simulink model "PMSM_FOC_Tractio"  (R2019b)
settings: Solver=FixedStepAuto  StartTime=0.0  StopTime=10  RelTol=1e-3
model workspace (MAT data in the model file):
  wc = Simulink.Parameter
  wc.DataType = 'auto'
  wc.Dimensions = [0 0]
values from neighbouring files (symbols this model uses):
  Cosine_table = 1.0 0.99999529 0.99999058 0.99998587 0.99998116 0.99996704 0.99995291 0.99993885 0.99992472 0.99990118 0.99987763 0.99985409 0.9998306 0.99979764 0.99976468 0.99973178 0.99969882 0.99965644 0.99961412 0.99957174 0.99952942 0.99947762 0.99942589 0.99937415 0.99932235 0.9992612 0.99920005 0.99913889 0.99907768 0.99900717 0.99893659 0.99886602 0.99879545 0.99871546 0.99863547 0.99855554 0.99847555 0.    [Hall_HFI_FOC_Data.sldd]
  Flux = 0.00529276    [Hall_HFI_FOC_Data.sldd]
  MTPA_id_table = 0.22889 0.23462678 0.23770036 0.2381243 0.23591207 0.23107713 0.2236329 0.21359272 0.20096992 0.18577772 0.16802935 0.14773798 0.12491672 0.099578641 0.071736768 0.041404068 0.0085934745 -0.026682133 -0.064409919 -0.10457709 -0.14717092 -0.1921787 -0.2395878 -0.28938559 -0.34155953 -0.39609709 -0.45298585 -0.51221335 -0.57376724 -0.63763517 -0.70380485 -0.77226412 -0.84300071 -0.91600245 -0.991257    [Hall_HFI_FOC_Data.sldd]
  MTPA_iq_table = -1.0417 -0.16083497 0.71926296 1.5985928 2.4771533 3.3549435 4.2319627 5.1082091 5.9836826 6.8583813 7.732305 8.6054525 9.4778223 10.349415 11.220228 12.090261 12.959513 13.827983 14.69567 15.562573 16.428694 17.294027 18.158575 19.022335 19.885307 20.747492 21.608887 22.469492 23.329306 24.188328 25.046556 25.903992 26.760633 27.616482 28.471533 29.325788 30.179247 31.031908 31.883772 32.734837 3    [Hall_HFI_FOC_Data.sldd]
  MTPA_Te_Max = 800.0    [Hall_HFI_FOC_Data.sldd]
  MTPA_Te_Min = 0.0    [Hall_HFI_FOC_Data.sldd]
  Sine_table = 0.0 0.0015339879 0.0030679768 0.0046019657 0.0061359555 0.0076698866 0.0092038177 0.010737749 0.012271681 0.013805497 0.015339312 0.016873131 0.018406944 0.019940587 0.021474229 0.023007872 0.024541514 0.026074925 0.027608337 0.029141748 0.03067516 0.032208283 0.033741407 0.035274528 0.036807653 0.038340431 0.039873205 0.04140598 0.042938754 0.04447113 0.046003502 0.047535874 0.049068246 0.0506001    [Hall_HFI_FOC_Data.sldd]
undefined symbols (not defined in the file or in its folder): CL_Param, ctrlParamsPI, DiscIntNeverNeededParam, Flux_weak, HFI, inverter, magnitude, OPL_Param, pmsm, sigbuilder_block, SMO, SVPWM
libraries: powerlib x22, fl_lib x18, simulink x7, nesl_utility x7, powerlib_meascontrol x3, dspstat3 x3, powerlib_extras x1, ee_lib x1
(part 1 of 4)
settings Model: Creator=jt  LastModifiedBy=Administrator
settings DataIOCC: LimitDataPoints=on  SaveFormat=Array  ReturnWorkspaceOutputs=off
settings OptimizationCC: DefaultParameterBehavior=Inlined  UseDivisionForNetSlopeComputation=on  GainParamInheritBuiltInType=on  UseFloatMulNetSlope=on  InlineInvariantSignals=on  PassReuseOutputArgsAs=Individual arguments  ZeroExternalMemoryAtStartup=off  ZeroInternalMemoryAtStartup=off  NoFixptDivByZeroProtection=on  EfficientFloat2IntCast=on  LifeSpan=1  OptimizeBlockOrder=speed  DifferentSizesBufferReuse=on  EfficientTunableParamExpr=on
settings DebuggingCC: AlgebraicLoopMsg=none  MaxConsecutiveZCsMsg=none  SolverPrmCheckMsg=warning  ParameterTunabilityLossMsg=error  AllowSymbolicDim=off  SFUnexpectedBacktrackingDiag=warning  SFNoUnconditionalDefaultTransitionDiag=warning  SFExecutionAtInitializationDiag=none  ArithmeticOperatorsInVariantConditions=warning
settings HardwareCC: ProdBitPerPointer=32  ProdBitPerSizeT=32  ProdBitPerPtrDiffT=32  ProdLargestAtomicInteger=Long  ProdLargestAtomicFloat=Double  ProdEndianess=BigEndian  ProdWordSize=32  ProdLongLongMode=on  ProdHWDeviceType=Freescale->32-bit PowerPC
settings ModelReferenceCC: PropagateSignalLabelsOutOfModel=off
settings SFSimCC: SimUseLocalCustomCode=off  SimParseCustomCode=off  MATLABDynamicMemAlloc=off  CustomCodeUndefinedFunction=UseInterfaceOnly
settings RTWCC: SystemTargetFile=ert.tlc  GenCodeOnly=on  TemplateMakefile=ert_default_tmf  GenerateReport=on  RTWUseLocalCustomCode=off  IncludeHyperlinkInReport=on  LaunchReport=on  GenerateTraceInfo=on  GenerateTraceReport=on  GenerateTraceReportSl=on  GenerateTraceReportSf=on  GenerateTraceReportEml=on  GenerateCodeMetricsReport=on
settings CodeAppCC: ForceParamTrailComments=on  IgnoreCustomStorageClasses=off  OperatorAnnotations=on  SimulinkDataObjDesc=on  SFDataObjDesc=on  CustomSymbolStrGlobalVar=rt$N$M  CustomSymbolStrType=$N$M  CustomSymbolStrFcn=$N$M$F  CustomSymbolStrMacro=$N$M  InsertBlockDesc=on
settings ERTTargetCC: GenerateSampleERTMain=on  IncludeMdlTerminateFcn=off  CombineSignalStateStructs=on  SupportNonInlinedSFcns=on  InlinedParameterPlacement=NonHierarchical  ERTCustomFileTemplate=example_file_process.tlc
settings ConfigComp: CovMetricSettings=dw  CovHtmlReporting=on  CovSaveCumulativeToWorkspaceVar=on  CovSaveSingleToWorkspaceVar=on  CovExternalEMLEnable=off  CovSFcnEnable=off
settings SimscapeCC: SimscapeNormalizeSystem=off

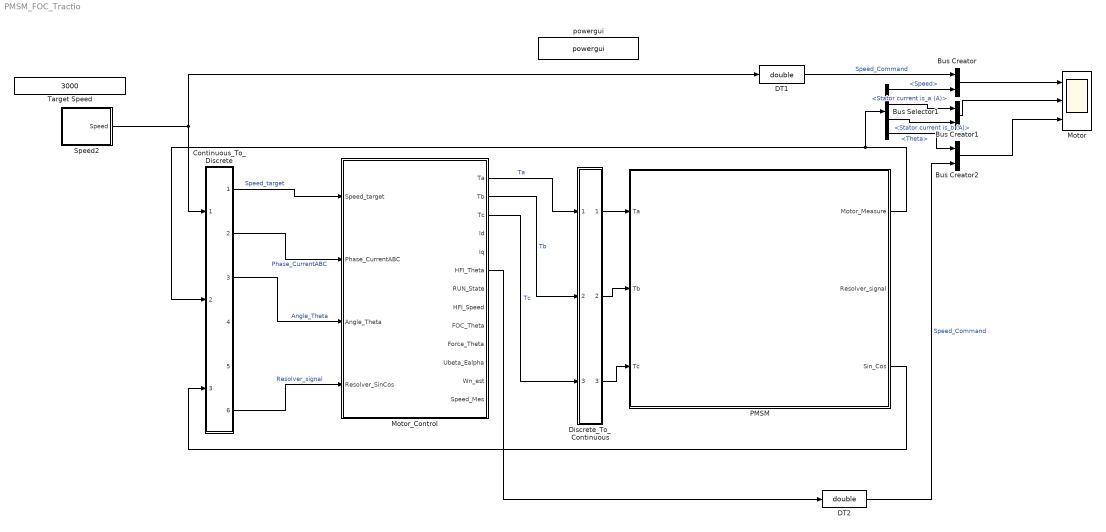
== system PMSM_FOC_Tractio ==
  Bus Creator : BusCreator  Inputs=2
  Bus Creator1 : BusCreator  Inputs=2
  Bus Creator2 : BusCreator  Inputs=2
  Bus Selector1 : BusSelector  OutputSignals=Speed,Stator current is_a (A),Stator current is_b (A),Theta
  Continuous_To_Discrete : Subsystem
      mask Display: fprintf('C/D')
  DT1 : DataTypeConversion  OutDataTypeStr=double
  DT2 : DataTypeConversion  OutDataTypeStr=double
  Discrete_To_Continuous : Subsystem  Description=""
      mask Display: fprintf('D/C')
  Motor : Scope  NumInputPorts=3
  Motor_Control : Subsystem  TreatAsAtomicUnit=on
  PMSM : Subsystem
      mask Display: image('$imagefile'); % Use "Edit Image" on toolstrip to change.
  Speed2 : Subsystem  Tag=STV Subsys  LoadFcn=sigbuilder_block('load');  StartFcn=sigbuilder_block('start');  StopFcn=sigbuilder_block('stop');  ClipboardFcn=sigbuilder_block('clipboard');  mask(Sigbuilder block){tuvar=[0:10]}
      mask help: Simulink:masks:SigbuilderBlock_MD
      mask init:
      | if ~strcmp(get_param(bdroot(gcbh),'SimulationStatus'),'stopped') tuvar = sigbuilder_block('maskInit'); end
      settings: CopyFcn=sigbuilder_block('copy');  DeleteFcn=sigbuilder_block('delete');  ModelCloseFcn=sigbuilder_block('modelClose');  PreSaveFcn=sigbuilder_block('preSave');  PauseFcn=sigbuilder_block('pause');  ContinueFcn=sigbuilder_block('continue');  NameChangeFcn=sigbuilder_block('namechange');  OpenFcn=sigbuilder_block('open',[48.5 0 906 449 ]);  CloseFcn=sigbuilder_block('close');
      mask Display: plot(0, 0, 100, 100,[2, 2, 32, 32, 2], [68, 8, 8, 68, 68],[32, 2], [38, 38], [32, 19, 2],[53, 60, 44], [32, 17, 17, 2],[16, 16, 31, 31]);txt = getActiveGroup(gcbh);text(2, 100, txt,'verticalAlignment', 'top');
  Target Speed : Constant  Value=3000
  powergui : powerlib/powergui  Priority=1  SimulationMode=Discrete  SampleTime=1e-5  frequency=60  Iterations=50  frequencyindice=0  Pbase=100e6  ErrMax=1e-4  UnitsV=kV  UnitsW=MW  buscounter=0  FunctionMessages=off  echomessages=off  EnableUseOfTLC=off  CurrentSourceSwitches=off  DisableSnubberDevices=off  DisableRonSwitches=off  DisableVfSwitches=off  DisplayEquations=off  AutomaticDiscreteSolvers=off  SolverType=Tustin  Interpol=off  ExternalGateDelay=off  methode=off  Ts=0  x0status=blocks  SPID=off  SwTol=0  HookPort=off  NonlinearTolerance=1e-4  nMaxIteration=100  ContinueOnMaxIteration=off  RestoreLinks=warning  ResistiveCurrentMeasurement=off  Frange=[0:2:500]  Ylog=off  Xlog=on  ShowGrid=off  save=off  variable=ZData  structure=0  ZoomFFT=on  StartTime=0.0  cycles=1  DisplayStyle=1  fundamental=60  FreqAxis=off  MaxFrequency=1000  frequencyindicesteady=1  RmsSteady=1  display=off
      settings: SourceProductName=Simscape Electrical
  wires:
  Discrete_To_Continuous/1(T1) -> PMSM/1(Ta)
  Discrete_To_Continuous/2(T2) -> PMSM/2(Tb)
  Discrete_To_Continuous/3(T3) -> PMSM/3(Tc)
  PMSM/1(Motor_Measure) -> Continuous_To_Discrete/2(Motor_Measurements), Bus Selector1/1
  Continuous_To_Discrete/1(Speed_target) -> Motor_Control/1(Speed_target)  "Speed_target"
  Continuous_To_Discrete/3(Theta) -> Motor_Control/3(Angle_Theta)  "Angle_Theta"
  Motor_Control/1(Ta) -> Discrete_To_Continuous/1(Ta)  "Ta"
  Motor_Control/2(Tb) -> Discrete_To_Continuous/2(Tb)  "Tb"
  Motor_Control/3(Tc) -> Discrete_To_Continuous/3(Tc)  "Tc"
  Bus Selector1/1 -> Bus Creator/2  "<Speed>"
  Bus Creator/1 -> Motor/1
  Bus Selector1/2 -> Bus Creator1/1  "<Stator current is_a (A)>"
  Bus Selector1/3 -> Bus Creator1/2  "<Stator current is_b (A)>"
  Bus Creator1/1 -> Motor/2
  Speed2/1(Speed) -> DT1/1, Continuous_To_Discrete/1(Speed_Command)
  DT1/1 -> Bus Creator/1  "Speed_Command"
  Continuous_To_Discrete/6(Resolver_measured) -> Motor_Control/4(Resolver_SinCos)  "Resolver_signal"
  PMSM/3(Sin_Cos) -> Continuous_To_Discrete/3(Sin_Cos)
  Continuous_To_Discrete/2(Phase_CurrentABC) -> Motor_Control/2(Phase_CurrentABC)  "Phase_CurrentABC"
  Bus Selector1/4 -> Bus Creator2/1  "<Theta>"
  Motor_Control/6(HFI_Theta) -> DT2/1
  Bus Creator2/1 -> Motor/3
  DT2/1 -> Bus Creator2/2  "Speed_Command"

== system PMSM_FOC_Tractio/Continuous_To_Discrete ==
  note: Continuous To Discrete
  Speed_Command : Inport
  Motor_Measurements : Inport  Port=2
  Sin_Cos : Inport  Port=3
  Bus Selector1 : BusSelector  OutputSignals=Speed,Stator current is_a (A),Stator current is_b (A),Stator current is_c (A),Theta,Vabc
  Bus Selector2 : BusSelector  OutputSignals=Sin,Cos
  DT{1..6} (6 alike) : DataTypeConversion  OutDataTypeStr=single
  Mux1 : Mux  Inputs=2
  Mux2 : Mux  Inputs=3
  RT{1..5} (5 alike) : RateTransition  Integrity=off
  RT6 : RateTransition  Integrity=off  OutPortSampleTime=inverter.Ts
  Speed_target : Outport
  Phase_CurrentABC : Outport  Port=2  PortDimensions=3
  Theta : Outport  Port=3
  Vabc : Outport  Port=4
  Speed_val : Outport  Port=5
  Resolver_measured : Outport  Port=6
  wires:
  DT2/1 -> Speed_val/1  "Speed_Measure"
  DT1/1 -> Speed_target/1  "Speed_Command"
  RT2/1 -> DT2/1
  RT1/1 -> DT1/1
  RT3/1 -> DT3/1
  Motor_Measurements/1 -> Bus Selector1/1
  Speed_Command/1 -> RT1/1
  RT4/1 -> DT4/1
  DT4/1 -> Theta/1  "Theta_Angle"
  Bus Selector1/1 -> RT2/1  "<Speed>"
  Bus Selector1/5 -> RT4/1  "<Theta>"
  DT5/1 -> Vabc/1  "Vabc"
  RT5/1 -> DT5/1
  Bus Selector1/6 -> RT5/1  "<Vabc>"
  DT6/1 -> Resolver_measured/1  "Resolver"
  Sin_Cos/1 -> Bus Selector2/1
  Bus Selector2/1 -> Mux1/1  "<Sin>"
  Bus Selector2/2 -> Mux1/2  "<Cos>"
  Mux1/1 -> RT6/1
  RT6/1 -> DT6/1
  Bus Selector1/2 -> Mux2/1  "<Stator current is_a (A)>"
  Bus Selector1/4 -> Mux2/3  "<Stator current is_c (A)>"
  Bus Selector1/3 -> Mux2/2  "<Stator current is_b (A)>"
  Mux2/1 -> RT3/1
  DT3/1 -> Phase_CurrentABC/1  "Phase_CurrentABC"

== system PMSM_FOC_Tractio/Discrete_To_Continuous ==
  note: Discrete To Continuous
  Ta : Inport
  Tb : Inport  Port=2
  Tc : Inport  Port=3
  DT : DataTypeConversion
  DT1 : DataTypeConversion
  DT2 : DataTypeConversion
  RT : RateTransition  Integrity=off
  RT1 : RateTransition  Integrity=off
  RT2 : RateTransition  Integrity=off
  T1 : Outport
  T2 : Outport  Port=2
  T3 : Outport  Port=3
  wires:
  DT/1 -> RT/1
  Ta/1 -> DT/1  "Tabc"
  DT1/1 -> RT1/1
  Tb/1 -> DT1/1  "Tabc"
  DT2/1 -> RT2/1
  Tc/1 -> DT2/1  "Tabc"
  RT/1 -> T1/1  "Tabc"
  RT1/1 -> T2/1  "Tabc"
  RT2/1 -> T3/1  "Tabc"

== system PMSM_FOC_Tractio/Motor_Control ==
  Speed_target : Inport
  Phase_CurrentABC : Inport  Port=2  PortDimensions=3
  Angle_Theta : Inport  Port=3  OutMin=0  OutMax=2*pi
  Resolver_SinCos : Inport  Port=4  OutMin=0  OutMax=2*pi
  Motor_Control_Funtion : Subsystem
  Ta : Outport
  Tb : Outport  Port=2
  Tc : Outport  Port=3
  Id : Outport  Port=4
  Iq : Outport  Port=5
  HFI_Theta : Outport  Port=6
  RUN_State : Outport  Port=7
  HFI_Speed : Outport  Port=8
  FOC_Theta : Outport  Port=9
  Force_Theta : Outport  Port=10
  Ubeta_Ealpha : Outport  Port=11
  Wn_est : Outport  Port=12
  Speed_Mes : Outport  Port=13
  wires:
  Motor_Control_Funtion/2(Tb) -> Tb/1
  Motor_Control_Funtion/3(Tc) -> Tc/1
  Motor_Control_Funtion/1(Ta) -> Ta/1
  Motor_Control_Funtion/9(Id) -> Id/1
  Motor_Control_Funtion/10(Iq) -> Iq/1
  Motor_Control_Funtion/11(HFI_Theta) -> HFI_Theta/1
  Motor_Control_Funtion/12(RUN_State) -> RUN_State/1
  Motor_Control_Funtion/13(HFI_Speed) -> HFI_Speed/1
  Motor_Control_Funtion/4(FOC_Theta) -> FOC_Theta/1
  Motor_Control_Funtion/5(Force_Theta) -> Force_Theta/1
  Motor_Control_Funtion/6(Ubeta_Ealpha) -> Ubeta_Ealpha/1
  Motor_Control_Funtion/7(Wn_est) -> Wn_est/1
  Motor_Control_Funtion/8(Speed_Mes) -> Speed_Mes/1
  Speed_target/1 -> Motor_Control_Funtion/1(Speed_target)  "Speed_target"
  Phase_CurrentABC/1 -> Motor_Control_Funtion/2(Phase_CurrentABC)  "Phase_CurrentABC"
  Angle_Theta/1 -> Motor_Control_Funtion/3(Angle_Theta)  "Angle_Theta"
  Resolver_SinCos/1 -> Motor_Control_Funtion/4(Resolver_SinCos)  "Resolver_signal"

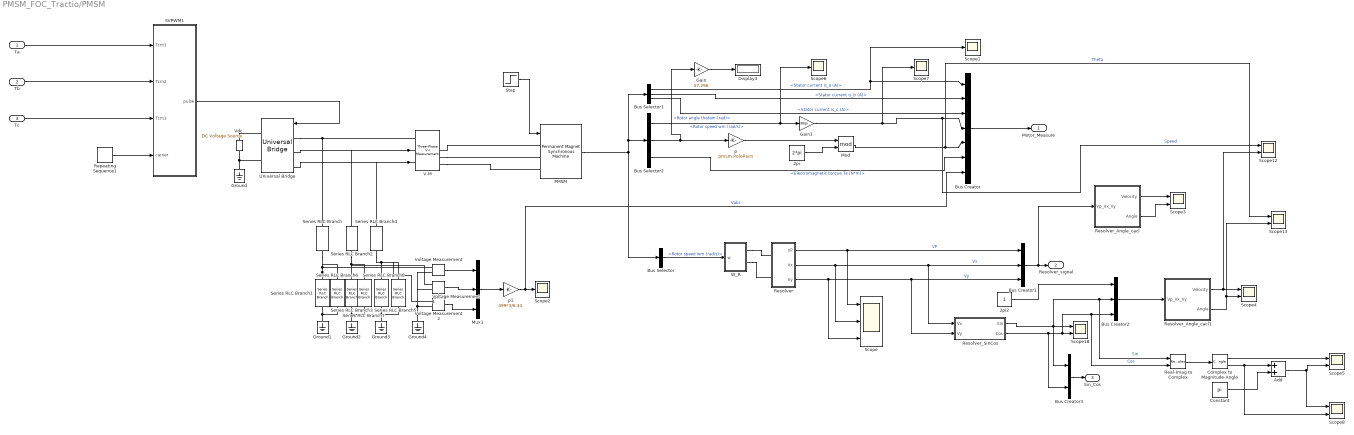
== system PMSM_FOC_Tractio/PMSM ==
  Ta : Inport
  Tb : Inport  Port=2
  Tc : Inport  Port=3
  2pi : Constant  Value=2*pi
  2pi2 : Constant
  Add : Sum
  Bus Creator : BusCreator  Inputs=7
  Bus Creator1 : BusCreator  Inputs=3
  Bus Creator2 : BusCreator  Inputs=3
  Bus Creator3 : BusCreator  Inputs=2
  Bus Selector : BusSelector  OutputSignals=Rotor speed wm (rad/s)
  Bus Selector1 : BusSelector  OutputSignals=Stator current is_a (A),Stator current is_b (A),Stator current is_c (A)
  Bus Selector2 : BusSelector  OutputSignals=Rotor speed wm (rad/s),Rotor angle thetam (rad),Electromagnetic torque Te (N*m)
  Complex to Magnitude-Angle : ComplexToMagnitudeAngle
  Constant : Constant  Value=pi
  Display3 : Display
  Gain : Gain  Gain=57.296
  Gain1 : Gain  Gain=30/pi  OutDataTypeStr=Inherit: Same as input  ParamDataTypeStr=Inherit: Same as input
  Ground{,1..4} (5 alike) : powerlib/Elements/Ground  LConnTagsString=a
      settings: SourceProductName=Simscape Electrical
  Mod : Math  Operator=mod  SignedPower=off  SaturateOnIntegerOverflow=on
  Mux1 : Mux  Inputs=3
  PMSM : powerlib/Machines/Permanent Magnet Synchronous Machine  NbPhases=3  FluxDistribution=Sinusoidal  RotorType=Salient-pole  MechanicalLoad=Torque Tm  PresetModel=No  ShowDetailedParameters=on  MeasurementBus=off  Resistance=pmsm.StatorPhaseResistance  Inductance=8.5e-3  dqInductances=[pmsm.InductanceLd pmsm.InductanceLq]  La=0.015  MachineConstant=Flux linkage established by magnets (V.s)  Flux=pmsm.FluxLinkage  VoltageCst=11.3137  TorqueCst=0.093564  Flat=120  Mechanical=[1e-4 0 pmsm.PolePairs 0]  PolePairs=3  InitialConditions=[0,30,0,0]  InitialConditions5ph=[0 0 0 0 0 0]  RefAngle=Aligned with phase A axis (original Park)  IterativeDiscreteModel=Trapezoidal non iterative  TsBlock=-1  TsPowergui=0
  Real-Imag to Complex : RealImagToComplex
  Repeating Sequence1 : simulink/Sources/Repeating Sequence  rep_seq_t=[0 inverter.Ts/2 inverter.Ts]  rep_seq_y=[0 0.00005*200000000 0]
  Resolver : Subsystem
  Resolver_Angle_cacl : Subsystem  TreatAsAtomicUnit=on
      settings: RTWSystemCode=Nonreusable function  RTWFcnNameOpts=Use subsystem name  RTWFileNameOpts=Use subsystem name  FunctionInterfaceSpec=Allow arguments
  Resolver_Angle_cacl1 : Subsystem  TreatAsAtomicUnit=on
      settings: RTWSystemCode=Nonreusable function  RTWFcnNameOpts=Use subsystem name  RTWFileNameOpts=Use subsystem name  FunctionInterfaceSpec=Allow arguments
  Resolver_SinCos : Subsystem
  SVPWM1 : Subsystem  TreatAsAtomicUnit=on
  Scope : Scope  NumInputPorts=3
  Scope{1..2,6..7} (4 alike) : Scope
  Scope{3..5,8,12..13,18} (7 alike) : Scope  NumInputPorts=2
  Series RLC Branch : powerlib/Elements/Series RLC Branch  LConnTagsString=__new0  RConnTagsString=__new0  BranchType=R  Resistance=499*1000*3  Inductance=1e-3  SetiL0=off  InitialCurrent=0  Capacitance=1e-6  Setx0=off  InitialVoltage=0  Measurements=None
      settings: SourceProductName=Simscape Electrical
  Series RLC Branch1 : powerlib/Elements/Series RLC Branch  LConnTagsString=__new0  RConnTagsString=__new0  BranchType=R  Resistance=6.34*1000  Inductance=1e-3  SetiL0=off  InitialCurrent=0  Capacitance=1e-6  Setx0=off  InitialVoltage=0  Measurements=None
      settings: SourceProductName=Simscape Electrical
  Series RLC Branch2 : powerlib/Elements/Series RLC Branch  LConnTagsString=__new0  RConnTagsString=__new0  BranchType=R  Resistance=499*3*1000  Inductance=1e-3  SetiL0=off  InitialCurrent=0  Capacitance=1e-6  Setx0=off  InitialVoltage=0  Measurements=None
      settings: SourceProductName=Simscape Electrical
  Series RLC Branch3 : powerlib/Elements/Series RLC Branch  LConnTagsString=__new0  RConnTagsString=__new0  BranchType=R  Resistance=6.34*1000  Inductance=1e-3  SetiL0=off  InitialCurrent=0  Capacitance=1e-6  Setx0=off  InitialVoltage=0  Measurements=None
      settings: SourceProductName=Simscape Electrical
  Series RLC Branch4 : powerlib/Elements/Series RLC Branch  LConnTagsString=__new0  RConnTagsString=__new0  BranchType=R  Resistance=499*3*1000  Inductance=1e-3  SetiL0=off  InitialCurrent=0  Capacitance=1e-6  Setx0=off  InitialVoltage=0  Measurements=None
      settings: SourceProductName=Simscape Electrical
  Series RLC Branch5 : powerlib/Elements/Series RLC Branch  LConnTagsString=__new0  RConnTagsString=__new0  BranchType=R  Resistance=6.34*1000  Inductance=1e-3  SetiL0=off  InitialCurrent=0  Capacitance=1e-6  Setx0=off  InitialVoltage=0  Measurements=None
      settings: SourceProductName=Simscape Electrical
  Series RLC Branch6 : powerlib/Elements/Series RLC Branch  LConnTagsString=__new0  RConnTagsString=__new0  BranchType=C  Resistance=6.34  Inductance=1e-3  SetiL0=off  InitialCurrent=0  Capacitance=0.047/1000000  Setx0=off  InitialVoltage=0  Measurements=None
      settings: SourceProductName=Simscape Electrical
  Series RLC Branch7 : powerlib/Elements/Series RLC Branch  LConnTagsString=__new0  RConnTagsString=__new0  BranchType=C  Resistance=6.34  Inductance=1e-3  SetiL0=off  InitialCurrent=0  Capacitance=0.047/1000000  Setx0=off  InitialVoltage=0  Measurements=None
      settings: SourceProductName=Simscape Electrical
  Series RLC Branch8 : powerlib/Elements/Series RLC Branch  LConnTagsString=__new0  RConnTagsString=__new0  BranchType=C  Resistance=6.34  Inductance=1e-3  SetiL0=off  InitialCurrent=0  Capacitance=0.047/1000000  Setx0=off  InitialVoltage=0  Measurements=None
      settings: SourceProductName=Simscape Electrical
  Step : Step  Time=1.5  After=0.05  SampleTime=0
  Universal Bridge : powerlib/Power Electronics/Universal Bridge  Arms=3  SnubberResistance=1e5  SnubberCapacitance=inf  Device=IGBT / Diodes  Ron=1e-3  Lon=0  ForwardVoltages="[  0  0  ]"  ForwardVoltage=0  GTOparameters=[ 10e-6 , 20e-6 ]  IGBTparameters=[ 1e-6 , 2e-6 ]  Measurements=None  Measurements_2=None  converterType=Rectifier
      settings: SourceProductName=Simscape Electrical
  V-M : powerlib/Measurements/Three-Phase V-I Measurement  VoltageMeasurement=phase-to-ground  SetLabelV=off  LabelV=Vabc  Vpu=off  VpuLL=off  CurrentMeasurement=yes  SetLabelI=off  LabelI=Iabc  Ipu=off  Pbase=100e6  Vbase=500e3  OutputType=Complex  PhasorSimulation=off  PSBequivalent=0
      settings: SourceProductName=Simscape Electrical
  "Vdc " : powerlib/Electrical Sources/DC Voltage Source  Amplitude=inverter.BusVoltage  Measurements=None
      settings: SourceProductName=Simscape Electrical
  Voltage Measurement : powerlib/Measurements/Voltage Measurement  PhasorSimulation=off  OutputType=Complex  PSBequivalent=0
      settings: SourceProductName=Simscape Electrical
  Voltage Measurement1 : powerlib/Measurements/Voltage Measurement  PhasorSimulation=off  OutputType=Complex  PSBequivalent=0
      settings: SourceProductName=Simscape Electrical
  Voltage Measurement2 : powerlib/Measurements/Voltage Measurement  PhasorSimulation=off  OutputType=Complex  PSBequivalent=0
      settings: SourceProductName=Simscape Electrical
  W_R : Subsystem
  p : Gain  Gain=pmsm.PolePairs  OutDataTypeStr=Inherit: Same as input  ParamDataTypeStr=Inherit: Same as input
  p1 : Gain  Gain=499*3/6.34  OutDataTypeStr=Inherit: Same as input  ParamDataTypeStr=Inherit: Same as input
  Motor_Measure : Outport
  Resolver_signal : Outport  Port=2
  Sin_Cos : Outport  Port=3
  wires:
  Repeating Sequence1/1 -> SVPWM1/4(carrier)
  SVPWM1/1(pulse) -> Universal Bridge/1
  Mod/1 -> Scope13/1, Bus Creator/5  "Theta"
  p1/1 -> Bus Creator/7, Scope2/1  "Vabc"
  Voltage Measurement2/1 -> Mux1/3
  Voltage Measurement/1 -> Mux1/1
  Mux1/1 -> p1/1
  2pi/1 -> Mod/2
  Voltage Measurement1/1 -> Mux1/2
  p/1 -> Mod/1
  Bus Selector2/2 -> Gain/1, p/1  "<Rotor angle thetam (rad)>"
  Bus Selector1/1 -> Scope1/1, Bus Creator/1  "<Stator current is_a (A)>"
  Bus Selector2/3 -> Bus Creator/6  "<Electromagnetic torque Te (N*m)>"
  Bus Selector1/2 -> Bus Creator/2  "<Stator current is_b (A)>"
  Bus Selector2/1 -> Scope6/1, Gain1/1  "<Rotor speed wm (rad/s)>"
  PMSM/1 -> Bus Selector2/1, Bus Selector1/1, Bus Selector/1
  Gain1/1 -> Scope7/1, Scope12/1, Bus Creator/4  "Speed"
  Bus Creator/1 -> Motor_Measure/1
  Ta/1 -> SVPWM1/1(Tcm1)
  Tb/1 -> SVPWM1/2(Tcm2)
  Tc/1 -> SVPWM1/3(Tcm3)
  Step/1 -> PMSM/1
  Bus Selector/1 -> W_R/1(w)  "<Rotor speed wm (rad/s)>"
  Resolver/2(Vx) -> Scope/2, Resolver_SinCos/1(Vx), Bus Creator1/2  "Vx"
  Resolver/3(Vy) -> Scope/3, Resolver_SinCos/2(Vy), Bus Creator1/3  "Vy"
  Bus Creator1/1 -> Resolver_Angle_cacl/1(Vp_Vx_Vy), Resolver_signal/1
  Resolver_Angle_cacl/1(Velocity) -> Scope3/1
  Resolver_Angle_cacl/2(Angle) -> Scope3/2
  Resolver_Angle_cacl1/2(Angle) -> Scope13/2, Scope4/2
  Resolver_Angle_cacl1/1(Velocity) -> Scope12/2, Scope4/1
  Bus Creator2/1 -> Resolver_Angle_cacl1/1(Vp_Vx_Vy)
  Real-Imag to Complex/1 -> Complex to Magnitude-Angle/1
  Complex to Magnitude-Angle/1 -> Scope5/1
  Resolver_SinCos/2(Cos) -> Bus Creator3/2, Real-Imag to Complex/2, Bus Creator2/3, Scope18/2  "Cos"
  Resolver_SinCos/1(Sin) -> Bus Creator3/1, Real-Imag to Complex/1, Bus Creator2/2, Scope18/1  "Sin"
  2pi2/1 -> Bus Creator2/1
  Resolver/1(VP) -> Scope/1, Bus Creator1/1  "VP"
  Bus Creator3/1 -> Sin_Cos/1
  Complex to Magnitude-Angle/2 -> Scope8/2, Add/1
  Add/1 -> Scope8/1, Scope5/2
  Constant/1 -> Add/2
  Bus Selector1/3 -> Bus Creator/3  "<Stator current is_c (A)>"
  Gain/1 -> Display3/1
  connections:
  "Vdc "/RConn1 -- Universal Bridge/RConn1
  Universal Bridge/RConn2 -- "Vdc "/LConn1 -- Ground/LConn1
  Series RLC Branch/RConn1 -- Universal Bridge/LConn1 -- V-M/LConn1
  V-M/LConn2 -- Universal Bridge/LConn2 -- Series RLC Branch2/RConn1
  V-M/LConn3 -- Universal Bridge/LConn3 -- Series RLC Branch4/RConn1
  Series RLC Branch8/RConn1 -- Series RLC Branch5/RConn1 -- Ground3/LConn1
  Ground4/LConn1 -- Voltage Measurement2/LConn2 -- Voltage Measurement/LConn2 -- Voltage Measurement1/LConn2
  Series RLC Branch2/LConn1 -- Series RLC Branch7/LConn1 -- Voltage Measurement1/LConn1 -- Series RLC Branch3/LConn1
  Series RLC Branch4/LConn1 -- Voltage Measurement2/LConn1 -- Series RLC Branch8/LConn1 -- Series RLC Branch5/LConn1
  Series RLC Branch6/RConn1 -- Series RLC Branch1/RConn1 -- Ground1/LConn1
  Series RLC Branch1/LConn1 -- Voltage Measurement/LConn1 -- Series RLC Branch/LConn1 -- Series RLC Branch6/LConn1
  Series RLC Branch7/RConn1 -- Series RLC Branch3/RConn1 -- Ground2/LConn1
  V-M/RConn1 -- PMSM/LConn1
  V-M/RConn2 -- PMSM/LConn2
  V-M/RConn3 -- PMSM/LConn3
  W_R/RConn1 -- Resolver/LConn1
  W_R/RConn2 -- Resolver/LConn2

== system PMSM_FOC_Tractio/Speed2 ==
  Demux : Demux  Tag=STV Demux  Outputs=1
  FromWs : FromWorkspace  Tag=STV FromWs  VariableName=tuvar  SampleTime=0
      SigBuilderData=|
      | common.afterFinalStr = 'Extrapolate'
      | common.sampleTime = 0
      | dataSet.timeRange = [0 10]
      | dataSet.name = '转速给定'
      | sbobj.Groups.Name = '转速给定'
      | sbobj.Groups.Signals.Name = 'Speed'
      | sbobj.Groups.Signals.XData = [0 2 10]
      | sbobj.Groups.Signals.YData = [0 995 995]
  Speed : Outport  Tag=STV Outport  VectorParamsAs1DForOutWhenUnconnected=off
  wires:
  Demux/1 -> Speed/1
  FromWs/1 -> Demux/1

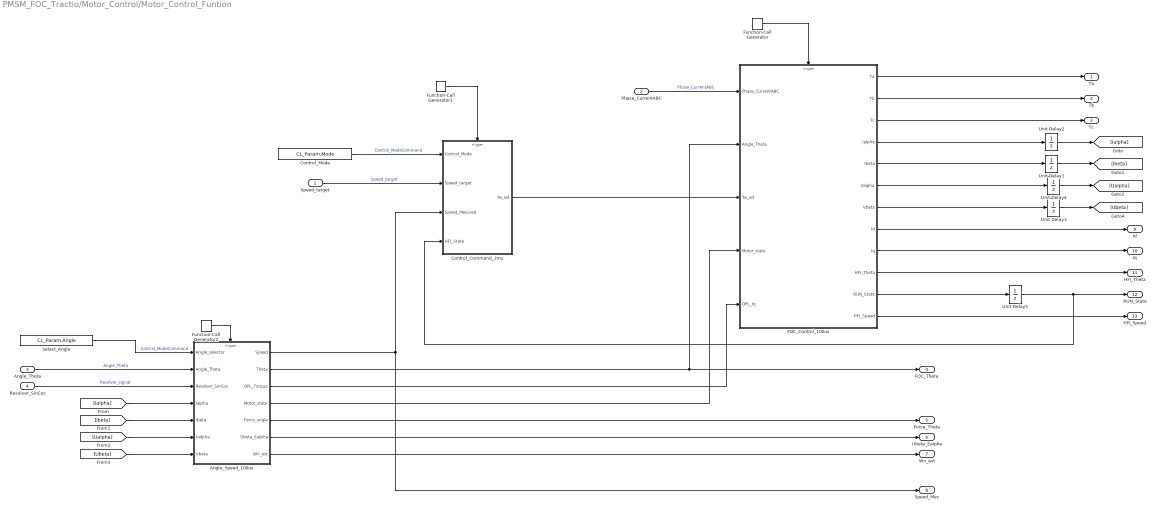
== system PMSM_FOC_Tractio/Motor_Control/Motor_Control_Funtion ==
  Speed_target : Inport
  Phase_CurrentABC : Inport  Port=2  PortDimensions=3
  Angle_Theta : Inport  Port=3  OutMin=0  OutMax=2*pi
  Resolver_SinCos : Inport  Port=4  OutMin=0  OutMax=2*pi
  Angle_Speed_100us : Subsystem
      settings: RTWSystemCode=Nonreusable function  RTWFcnNameOpts=Use subsystem name  RTWFileNameOpts=Use subsystem name
  Control_Command_2ms : Subsystem  TreatAsAtomicUnit=on
      settings: RTWSystemCode=Nonreusable function  RTWFcnNameOpts=Use subsystem name  RTWFileNameOpts=Use subsystem name  FunctionInterfaceSpec=Allow arguments
  Control_Mode : Constant  Value=CL_Param.Mode
  FOC_Control_100us : Subsystem  TreatAsAtomicUnit=on
      settings: RTWSystemCode=Nonreusable function  RTWFcnNameOpts=Use subsystem name  RTWFileNameOpts=Use subsystem name  FunctionInterfaceSpec=Allow arguments
  Function-Call Generator : simulink/Ports & Subsystems/Function-Call Generator  sample_time=inverter.Ts  numberOfIterations=1
  Function-Call Generator1 : simulink/Ports & Subsystems/Function-Call Generator  sample_time=inverter.Speed_PI_T  numberOfIterations=1
  Function-Call Generator2 : simulink/Ports & Subsystems/Function-Call Generator  sample_time=inverter.Ts  numberOfIterations=1
  Select_Angle : Constant  Value=CL_Param.Angle
  Unit Delay{1..5} (5 alike) : UnitDelay  SampleTime=-1  HasFrameUpgradeWarning=on
  Ta : Outport
  Tb : Outport  Port=2
  Tc : Outport  Port=3
  FOC_Theta : Outport  Port=4
  Force_Theta : Outport  Port=5
  Ubeta_Ealpha : Outport  Port=6
  Wn_est : Outport  Port=7
  Speed_Mes : Outport  Port=8
  Id : Outport  Port=9
  Iq : Outport  Port=10
  HFI_Theta : Outport  Port=11
  RUN_State : Outport  Port=12
  HFI_Speed : Outport  Port=13
  wires:
  FOC_Control_100us/7(Vbeta) -> Unit Delay3/1
  FOC_Control_100us/10(HFI_Theta) -> HFI_Theta/1
  Unit Delay5/1 -> Control_Command_2ms/4(HFI_State), RUN_State/1
  FOC_Control_100us/12(HFI_Speed) -> HFI_Speed/1
  FOC_Control_100us/5(Ibeta) -> Unit Delay1/1
  [Ialpha] -> Angle_Speed_100us/4(Ialpha)
  Angle_Speed_100us/6(Ubeta_Ealpha) -> Ubeta_Ealpha/1
  Angle_Speed_100us/2(Theta) -> FOC_Theta/1, FOC_Control_100us/2(Angle_Theta)
  FOC_Control_100us/4(Ialpha) -> Unit Delay2/1
  Resolver_SinCos/1 -> Angle_Speed_100us/3(Resolver_SinCos)  "Resolver_signal"
  Control_Command_2ms/1(Te_ref) -> FOC_Control_100us/3(Te_ref)
  FOC_Control_100us/9(Iq) -> Iq/1
  Function-Call Generator1/1 -> Control_Command_2ms/Trigger
  Angle_Speed_100us/7(Wn_est) -> Wn_est/1
  [Ibeta] -> Angle_Speed_100us/5(Ibeta)
  FOC_Control_100us/6(Valpha) -> Unit Delay4/1
  Control_Mode/1 -> Control_Command_2ms/1(Control_Mode)  "Control_ModeCommand"
  FOC_Control_100us/8(Id) -> Id/1
  Angle_Speed_100us/4(Motor_state) -> FOC_Control_100us/4(Motor_state)
  Unit Delay4/1 -> [Ualpha]
  Unit Delay3/1 -> [Ubeta]
  Angle_Theta/1 -> Angle_Speed_100us/2(Angle_Theta)  "Angle_Theta"
  [Ubeta] -> Angle_Speed_100us/7(Ubeta)
  Angle_Speed_100us/5(Force_angle) -> Force_Theta/1
  Angle_Speed_100us/3(OPL_Torque) -> FOC_Control_100us/5(OPL_Iq)
  Function-Call Generator/1 -> FOC_Control_100us/Trigger
  FOC_Control_100us/11(RUN_State) -> Unit Delay5/1
  Phase_CurrentABC/1 -> FOC_Control_100us/1(Phase_CurrentABC)  "Phase_CurrentABC"
  FOC_Control_100us/3(Tc) -> Tc/1
  Select_Angle/1 -> Angle_Speed_100us/1(Angle_selector)  "Control_ModeCommand"
  Speed_target/1 -> Control_Command_2ms/2(Speed_target)  "Speed_target"
  Angle_Speed_100us/1(Speed) -> Control_Command_2ms/3(Speed_Mesured), Speed_Mes/1
  [Ualpha] -> Angle_Speed_100us/6(Ualpha)
  Unit Delay1/1 -> [Ibeta]
  FOC_Control_100us/2(Tb) -> Tb/1
  FOC_Control_100us/1(Ta) -> Ta/1
  Unit Delay2/1 -> [Ialpha]
  Function-Call Generator2/1 -> Angle_Speed_100us/Trigger

== system PMSM_FOC_Tractio/PMSM/Resolver ==
  Friction1 : fl_lib/Mechanical/Rotational Elements/Rotational Friction  brkwy_trq=25 N*m  brkwy_vel=0.1 rad/s  Col_trq=20 N*m  visc_coef=0.1 N*m/(rad/s)  w_specify=off  w_priority=None  w=0 rad/s  w_nominal_specify=off  w_nominal_unit=rad/s  w_nominal_value=1  t_specify=off  t_priority=None  t=0 N*m  t_nominal_specify=off  t_nominal_unit=N*m  t_nominal_value=1
      settings: SourceProductName=Simscape
  Ideal Torque Sensor : fl_lib/Mechanical/Mechanical Sensors/Ideal Torque Sensor
  Meas Vxy : Subsystem
  Mechanical Rotational Reference2 : fl_lib/Mechanical/Rotational Elements/Mechanical Rotational Reference
  Motor & load inertia1 : fl_lib/Mechanical/Rotational Elements/Inertia  inertia=1e-4 kg*m^2  w_specify=on  w_priority=High  w=0 rpm  w_nominal_specify=off  w_nominal_unit=rad/s  w_nominal_value=1  t_specify=off  t_priority=High  t=0 N*m  t_nominal_specify=off  t_nominal_unit=N*m  t_nominal_value=1
  PS-Simulink Converter2 : nesl_utility/PS-Simulink Converter  PhysicalDomain=network_engine_domain  SubClassName=ps_output  LeftPortType=input  RightPortType=output  PseudoPeriodic=off  Frequencies=[]  Unit=N*m  AffineConversion=off
  Resolver : ee_lib/Sensors & Transducers/Resolver  parameterization=1  ratio=0.5  Rr=70 Ohm  Rs=180 Ohm  Xr=100 Ohm  Xs=300 Ohm  omega=10 kHz  Lr=0.0016 H  Ls=0.0048 H  k=0.35  N=pmsm.PolePairs  theta_specify=off  theta_priority=High  theta=0 deg  theta_nominal_specify=off  theta_nominal_unit=deg  theta_nominal_value=1
      settings: SourceProductName=Simscape Electrical  SourceProductBaseCode=PS  InternalSimscapePortConfiguration="{\"Bottom\":[],\"Left\":[{\"id\":\"p1\",\"label\":\"p1\",\"type\":\"foundation.electrical.electrical\"},{\"id\":\"p2\",\"label\":\"p2\",\"type\":\"foundation.electrical.electrical\"},{\"id\":\"R\",\"label\":\"R\",\"type\":\"foundation.mechanical.rotational.rotational\"},{\"id\":\"C\",\"label\":\"C\",\"type\":\"foundation.mechanical.rotational.rotational\"}],\"Right\":[{\"id\":\"x1\",\"label\":\"x1\",\"type\":\"foundation.electrical.electrical\"},{\"id\":\"x2\",\"label\":\"x2\",\"type\":\"foundation.electrical.electrical\"},{\"id\":\"y1\",\"label\":\"y1\",\"type\":\"foundation.electrical.electrical\"},{\"id\":\"y2\",\"label\":\"y2\",\"type\":\"foundation.electrical.electrical\"}],\"Top\":[]}"
  Scope : Scope  NumInputPorts=2
  Scope1 : Scope
  Solver Configuration : nesl_utility/Solver Configuration  PhysicalDomain=network_engine_domain  SubClassName=solver  LeftPortType=input  RightPortType=generic  Tones=[]  Harmonics=[]  SimulateNoise=off  Profile=off  UseLocalSampling=off  EnableSwitchedLinearOptims=on  FrequencyDomain=off  UseCCode=off  RelTol=0.001  AbsTol=1e-06  MinStep=1e-09  ToWorkspace=off  RevertToSquareIcSolve=off  NumHomotopyIterations=100  PhasorMode=off  PhasorModeNumHarmonics=1  DoDC=on  ResidualTolerance=1e-5  UseLocalSolver=off  LocalSolverChoice=NE_PARTITIONING_ADVANCER  LocalSolverSampleTime=1e-5  DoFixedCost=off  MaxNonlinIter=10  MaxModeIter=2  LinearAlgebra=auto  EquationFormulation=NE_TIME_EF  DelaysMemoryBudget=1024  AutomaticFiltering=off  FilteringTimeConstant=0.001  PartitionStorageMethod=AS_NEEDED  PartitionMemoryBudget=1024  PartitionMethod=ROBUST
  Vp : Subsystem
  1L : PMIOPort  Side=Left
  2L : PMIOPort  Port=2  Side=Left
  VP : Outport  VectorParamsAs1DForOutWhenUnconnected=off
  Vx : Outport  Port=2  VectorParamsAs1DForOutWhenUnconnected=off
  Vy : Outport  Port=3  VectorParamsAs1DForOutWhenUnconnected=off
  tag scope: trqMotor=global
  wires:
  PS-Simulink Converter2/1 -> [trqMotor]
  Meas Vxy/1(Vx) -> Scope/1, Vx/1
  Vp/1(Vp) -> Scope1/1, VP/1
  Meas Vxy/2(Vy) -> Scope/2, Vy/1
  connections:
  Ideal Torque Sensor/RConn2 -- PS-Simulink Converter2/LConn1
  1L/RConn1 -- Ideal Torque Sensor/LConn1
  Friction1/RConn1 -- 2L/RConn1 -- Resolver/LConn4 -- Solver Configuration/RConn1 -- Mechanical Rotational Reference2/LConn1
  Friction1/LConn1 -- Ideal Torque Sensor/RConn1 -- Resolver/LConn3 -- Motor & load inertia1/LConn1
  Meas Vxy/LConn2 -- Resolver/RConn2
  Resolver/RConn1 -- Meas Vxy/LConn1
  Meas Vxy/LConn3 -- Resolver/RConn3
  Meas Vxy/LConn4 -- Resolver/RConn4
  Vp/RConn1 -- Resolver/LConn1
  Vp/RConn2 -- Resolver/LConn2

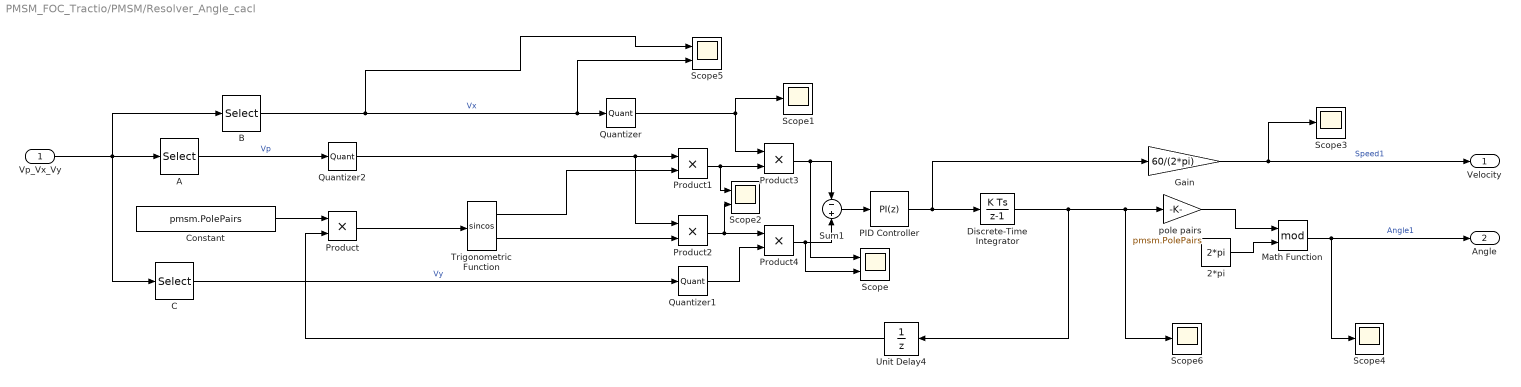
== system PMSM_FOC_Tractio/PMSM/Resolver_Angle_cacl ==
  Vp_Vx_Vy : Inport
  2*pi : Constant  Value=2*pi  OutDataTypeStr=single  SampleTime=-1
  A : Selector  IndexMode=Zero-based  InputPortWidth=3  IndexOptions=Index vector (dialog)  Indices=0  OutputSizes=1
  B : Selector  IndexMode=Zero-based  InputPortWidth=3  IndexOptions=Index vector (dialog)  Indices=1  OutputSizes=1
  C : Selector  IndexMode=Zero-based  InputPortWidth=3  IndexOptions=Index vector (dialog)  Indices=2  OutputSizes=1
  Constant : Constant  Value=pmsm.PolePairs  OutDataTypeStr=single  SampleTime=-1
  Discrete-Time Integrator : DiscreteIntegrator  SampleTime=-1  ICPrevOutput=DiscIntNeverNeededParam  ICPrevScaledInput=DiscIntNeverNeededParam
  Gain : Gain  Gain=60/(2*pi)
  Math Function : Math  Operator=mod  SaturateOnIntegerOverflow=on
  PID Controller : simulink/Continuous/PID Controller  Controller=PI  Form=Parallel  TimeDomain=Discrete-time  SampleTime=-1  IntegratorMethod=Forward Euler  FilterMethod=Forward Euler  ControllerParametersSource=internal  P=15  I=2.5e5  D=0  UseFilter=off  N=100  TunerSelectOption=Transfer Function Based (PID Tuner App)  InitialConditionSource=internal  InitialConditionForIntegrator=0  InitialConditionForFilter=0  DifferentiatorICPrevScaledInput=0  ExternalReset=none  TrackingMode=off  Kt=1  LimitOutput=off  UpperSaturationLimit=inf  LowerSaturationLimit=-inf  LinearizeAsGain=on  AntiWindupMode=none  Kb=1  POutMin=[]  POutMax=[]  IOutMin=[]  IOutMax=[]  DOutMin=[]  DOutMax=[]  NOutMin=[]  NOutMax=[]  SumOutMin=[]  SumOutMax=[]  SaturationOutMin=[]  SaturationOutMax=[]  PParamMin=[]  PParamMax=[]  IParamMin=[]  IParamMax=[]  DParamMin=[]  DParamMax=[]  NParamMin=[]  NParamMax=[]  KbParamMin=[]  KbParamMax=[]  KtParamMin=[]  KtParamMax=[]  KbOutMin=[]  KbOutMax=[]  KtOutMin=[]  KtOutMax=[]  IntegratorOutMin=[]  IntegratorOutMax=[]  FilterOutMin=[]  FilterOutMax=[]  SumI1OutMin=[]  SumI1OutMax=[]  SumI2OutMin=[]  SumI2OutMax=[]  SumI3OutMin=[]  SumI3OutMax=[]  SumI4OutMin=[]  SumI4OutMax=[]  SumDOutMin=[]  SumDOutMax=[]  DifferentiatorOutMin=[]  DifferentiatorOutMax=[]  FilterDiffOutCoefMin=[]  FilterDiffOutCoefMax=[]  ReciprocalOutMin=[]  ReciprocalOutMax=[]  SumDenOutMin=[]  SumDenOutMax=[]  SumNumOutMin=[]  SumNumOutMax=[]  DivideOutMin=[]  DivideOutMax=[]  IntegratorContinuousStateAttributes=''  IntegratorStateMustResolveToSignalObject=off  IntegratorRTWStateStorageClass=Auto  FilterContinuousStateAttributes=''  FilterStateMustResolveToSignalObject=off  FilterRTWStateStorageClass=Auto  ParallelPVariant=InternalParameters  IdealPVariant=Disabled  IVariant=InternalParameters  DVariant=Disabled  IntegratorVariant=Discrete  SatVariant=Disabled  AWVariant=Passthrough  PCopyVariant=Disabled  TRVariant=Disabled  FdbkBlocksVariant=Forward  IdealPFdbkVariant=Disabled  SatFdbkVariant=Disabled  DerivativeFilterVariant=Disabled  NVariant=Disabled  NCopyVariant=Disabled_SignalSpec  FilterICVariant=Disabled  IntegratorICVariant=InternalICs  ExternalResetVariant=Disabled  TRSumVariant=Passthrough  SumFdbkVariant=Disabled  SumVariant=Sum_PI
  Product : Product  OutDataTypeStr=single
  Product{1..4} (4 alike) : Product
  Quantizer : Quantizer  QuantizationInterval=1e-5
  Quantizer1 : Quantizer  QuantizationInterval=1e-5
  Quantizer2 : Quantizer  QuantizationInterval=1e-5
  Scope : Scope  NumInputPorts=2
  Scope{1,3..4,6} (4 alike) : Scope
  Scope2 : Scope  NumInputPorts=2
  Scope5 : Scope  NumInputPorts=2
  Sum1 : Sum  Inputs=-+
  Trigonometric Function : Trigonometry  Operator=sincos
  Unit Delay4 : UnitDelay  SampleTime=-1  HasFrameUpgradeWarning=on
  "pole pairs " : Gain  Gain=pmsm.PolePairs  OutDataTypeStr=single
  Velocity : Outport  VectorParamsAs1DForOutWhenUnconnected=off
  Angle : Outport  Port=2  VectorParamsAs1DForOutWhenUnconnected=off
  wires:
  Quantizer/1 -> Scope1/1, Product3/1
  Quantizer1/1 -> Product4/2
  Product2/1 -> Scope2/2, Product4/1
  Product4/1 -> Scope/2, Sum1/2
  Trigonometric Function/2 -> Product2/2
  Vp_Vx_Vy/1 -> C/1, B/1, A/1
  Unit Delay4/1 -> Product/2
  Sum1/1 -> PID Controller/1
  Product3/1 -> Scope/1, Sum1/1
  Constant/1 -> Product/1
  Quantizer2/1 -> Product2/1, Product1/1
  Product/1 -> Trigonometric Function/1
  Trigonometric Function/1 -> Product1/2
  Product1/1 -> Scope2/1, Product3/2
  Math Function/1 -> Angle/1, Scope4/1  "Angle1"
  Gain/1 -> Velocity/1, Scope3/1  "Speed1"
  Discrete-Time Integrator/1 -> Scope6/1, "pole pairs "/1, Unit Delay4/1
  "pole pairs "/1 -> Math Function/1
  PID Controller/1 -> Discrete-Time Integrator/1, Gain/1
  2*pi/1 -> Math Function/2
  A/1 -> Quantizer2/1  "Vp"
  B/1 -> Scope5/1, Quantizer/1, Scope5/2  "Vx"
  C/1 -> Quantizer1/1  "Vy"

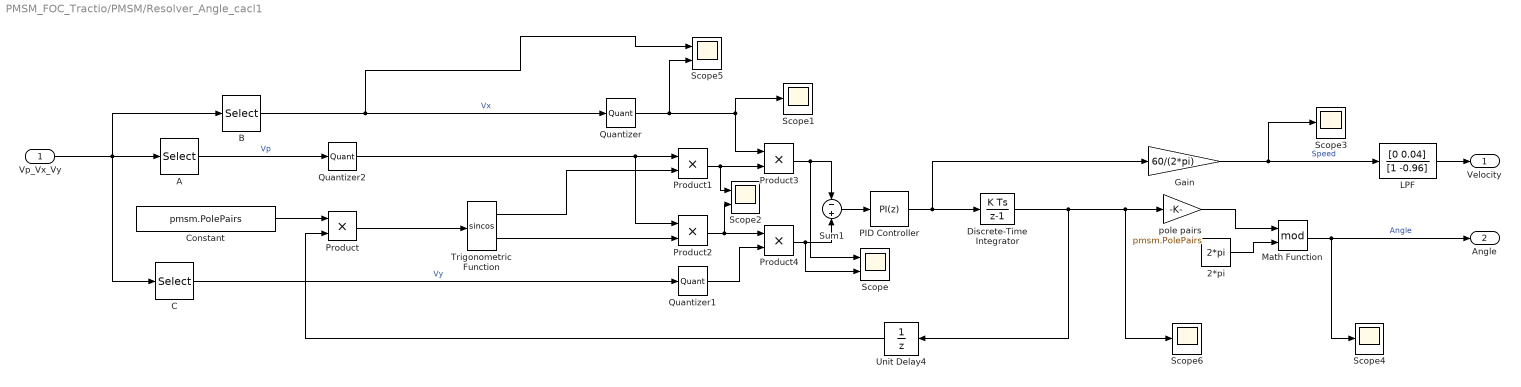
== system PMSM_FOC_Tractio/PMSM/Resolver_Angle_cacl1 ==
  Vp_Vx_Vy : Inport
  2*pi : Constant  Value=2*pi  OutDataTypeStr=single  SampleTime=-1
  A : Selector  IndexMode=Zero-based  InputPortWidth=3  IndexOptions=Index vector (dialog)  Indices=0  OutputSizes=1
  B : Selector  IndexMode=Zero-based  InputPortWidth=3  IndexOptions=Index vector (dialog)  Indices=1  OutputSizes=1
  C : Selector  IndexMode=Zero-based  InputPortWidth=3  IndexOptions=Index vector (dialog)  Indices=2  OutputSizes=1
  Constant : Constant  Value=pmsm.PolePairs  OutDataTypeStr=single  SampleTime=-1
  Discrete-Time Integrator : DiscreteIntegrator  SampleTime=-1  ICPrevOutput=DiscIntNeverNeededParam  ICPrevScaledInput=DiscIntNeverNeededParam
  Gain : Gain  Gain=60/(2*pi)
  LPF : DiscreteFilter  Numerator=[0 0.04]  Denominator=[1 -0.96]  SampleTime=inverter.Ts
  Math Function : Math  Operator=mod  SaturateOnIntegerOverflow=on
  PID Controller : simulink/Continuous/PID Controller  Controller=PI  Form=Parallel  TimeDomain=Discrete-time  SampleTime=-1  IntegratorMethod=Forward Euler  FilterMethod=Forward Euler  ControllerParametersSource=internal  P=120  I=2500  D=0  UseFilter=off  N=100  TunerSelectOption=Transfer Function Based (PID Tuner App)  InitialConditionSource=internal  InitialConditionForIntegrator=0  InitialConditionForFilter=0  DifferentiatorICPrevScaledInput=0  ExternalReset=none  TrackingMode=off  Kt=1  LimitOutput=off  UpperSaturationLimit=inf  LowerSaturationLimit=-inf  LinearizeAsGain=on  AntiWindupMode=none  Kb=1  POutMin=[]  POutMax=[]  IOutMin=[]  IOutMax=[]  DOutMin=[]  DOutMax=[]  NOutMin=[]  NOutMax=[]  SumOutMin=[]  SumOutMax=[]  SaturationOutMin=[]  SaturationOutMax=[]  PParamMin=[]  PParamMax=[]  IParamMin=[]  IParamMax=[]  DParamMin=[]  DParamMax=[]  NParamMin=[]  NParamMax=[]  KbParamMin=[]  KbParamMax=[]  KtParamMin=[]  KtParamMax=[]  KbOutMin=[]  KbOutMax=[]  KtOutMin=[]  KtOutMax=[]  IntegratorOutMin=[]  IntegratorOutMax=[]  FilterOutMin=[]  FilterOutMax=[]  SumI1OutMin=[]  SumI1OutMax=[]  SumI2OutMin=[]  SumI2OutMax=[]  SumI3OutMin=[]  SumI3OutMax=[]  SumI4OutMin=[]  SumI4OutMax=[]  SumDOutMin=[]  SumDOutMax=[]  DifferentiatorOutMin=[]  DifferentiatorOutMax=[]  FilterDiffOutCoefMin=[]  FilterDiffOutCoefMax=[]  ReciprocalOutMin=[]  ReciprocalOutMax=[]  SumDenOutMin=[]  SumDenOutMax=[]  SumNumOutMin=[]  SumNumOutMax=[]  DivideOutMin=[]  DivideOutMax=[]  IntegratorContinuousStateAttributes=''  IntegratorStateMustResolveToSignalObject=off  IntegratorRTWStateStorageClass=Auto  FilterContinuousStateAttributes=''  FilterStateMustResolveToSignalObject=off  FilterRTWStateStorageClass=Auto  ParallelPVariant=InternalParameters  IdealPVariant=Disabled  IVariant=InternalParameters  DVariant=Disabled  IntegratorVariant=Discrete  SatVariant=Disabled  AWVariant=Passthrough  PCopyVariant=Disabled  TRVariant=Disabled  FdbkBlocksVariant=Forward  IdealPFdbkVariant=Disabled  SatFdbkVariant=Disabled  DerivativeFilterVariant=Disabled  NVariant=Disabled  NCopyVariant=Disabled_SignalSpec  FilterICVariant=Disabled  IntegratorICVariant=InternalICs  ExternalResetVariant=Disabled  TRSumVariant=Passthrough  SumFdbkVariant=Disabled  SumVariant=Sum_PI
  Product : Product  OutDataTypeStr=single
  Product{1..4} (4 alike) : Product
  Quantizer : Quantizer  QuantizationInterval=1e-5
  Quantizer1 : Quantizer  QuantizationInterval=1e-5
  Quantizer2 : Quantizer  QuantizationInterval=1e-5
  Scope : Scope  NumInputPorts=2
  Scope{1,3..4,6} (4 alike) : Scope
  Scope2 : Scope  NumInputPorts=2
  Scope5 : Scope  NumInputPorts=2
  Sum1 : Sum  Inputs=-+
  Trigonometric Function : Trigonometry  Operator=sincos
  Unit Delay4 : UnitDelay  SampleTime=-1  HasFrameUpgradeWarning=on
  "pole pairs " : Gain  Gain=pmsm.PolePairs  OutDataTypeStr=single
  Velocity : Outport  VectorParamsAs1DForOutWhenUnconnected=off
  Angle : Outport  Port=2  VectorParamsAs1DForOutWhenUnconnected=off
  wires:
  Quantizer/1 -> Scope1/1, Product3/1, Scope5/2
  Quantizer1/1 -> Product4/2
  Product2/1 -> Scope2/2, Product4/1
  Product4/1 -> Scope/2, Sum1/2
  Trigonometric Function/2 -> Product2/2
  Vp_Vx_Vy/1 -> C/1, B/1, A/1
  Unit Delay4/1 -> Product/2
  Sum1/1 -> PID Controller/1
  Product3/1 -> Scope/1, Sum1/1
  Constant/1 -> Product/1
  Quantizer2/1 -> Product2/1, Product1/1
  Product/1 -> Trigonometric Function/1
  Trigonometric Function/1 -> Product1/2
  Product1/1 -> Scope2/1, Product3/2
  Math Function/1 -> Angle/1, Scope4/1  "Angle"
  Gain/1 -> LPF/1, Scope3/1  "Speed"
  Discrete-Time Integrator/1 -> Scope6/1, "pole pairs "/1, Unit Delay4/1
  "pole pairs "/1 -> Math Function/1
  PID Controller/1 -> Discrete-Time Integrator/1, Gain/1
  2*pi/1 -> Math Function/2
  A/1 -> Quantizer2/1  "Vp"
  B/1 -> Scope5/1, Quantizer/1  "Vx"
  C/1 -> Quantizer1/1  "Vy"
  LPF/1 -> Velocity/1

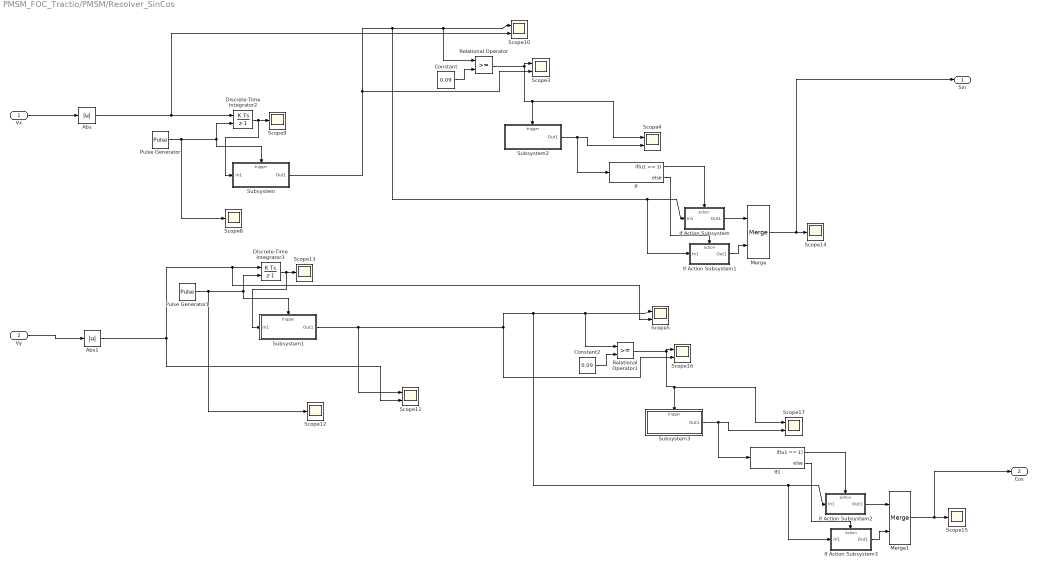
== system PMSM_FOC_Tractio/PMSM/Resolver_SinCos ==
  Vx : Inport
  Vy : Inport  Port=2
  Abs : Abs
  Abs1 : Abs
  Constant : Constant  Value=0.09
  Constant2 : Constant  Value=0.09
  Discrete-Time Integrator2 : DiscreteIntegrator  gainval=15625  ExternalReset=falling  SampleTime=-1  ICPrevOutput=DiscIntNeverNeededParam  ICPrevScaledInput=DiscIntNeverNeededParam
  Discrete-Time Integrator3 : DiscreteIntegrator  gainval=15625  ExternalReset=falling  SampleTime=-1  ICPrevOutput=DiscIntNeverNeededParam  ICPrevScaledInput=DiscIntNeverNeededParam
  If : If  IfExpression=u1 == 1
  If Action Subsystem : Subsystem  TreatAsAtomicUnit=on
  If Action Subsystem1 : Subsystem  TreatAsAtomicUnit=on
  If Action Subsystem2 : Subsystem  TreatAsAtomicUnit=on
  If Action Subsystem3 : Subsystem  TreatAsAtomicUnit=on
  If1 : If  IfExpression=u1 == 1
  Merge : Merge
  Merge1 : Merge
  Pulse Generator : DiscretePulseGenerator  PulseType=Time based  Period=inverter.Ts  PulseWidth=5
  Pulse Generator1 : DiscretePulseGenerator  PulseType=Time based  Period=inverter.Ts  PulseWidth=5
  Relational Operator : RelationalOperator  OutDataTypeStr=boolean  RndMeth=Simplest
  Relational Operator1 : RelationalOperator  OutDataTypeStr=boolean  RndMeth=Simplest
  Scope{3..5,10..11,16..17} (7 alike) : Scope  NumInputPorts=2
  Scope{8..9,12..15} (6 alike) : Scope
  Subsystem : Subsystem
  Subsystem1 : Subsystem
  Subsystem2 : Subsystem
  Subsystem3 : Subsystem
  Sin : Outport
  Cos : Outport  Port=2
  wires:
  Discrete-Time Integrator2/1 -> Subsystem/1(In1), Scope9/1
  Subsystem/1(Out1) -> If Action Subsystem1/1(In1), If Action Subsystem/1(In1), Relational Operator/1, Scope10/1, Scope3/2
  Subsystem2/1(Out1) -> If/1, Scope4/2
  Pulse Generator/1 -> Scope8/1, Discrete-Time Integrator2/2, Subsystem/Trigger
  If Action Subsystem2/1(Out1) -> Merge1/1
  If1/1 -> If Action Subsystem2/Action
  Relational Operator1/1 -> Scope17/1, Subsystem3/Trigger, Scope16/1
  Merge1/1 -> Cos/1, Scope15/1
  Constant2/1 -> Relational Operator1/2
  Subsystem3/1(Out1) -> If1/1, Scope17/2
  Abs1/1 -> Scope5/2, Discrete-Time Integrator3/1, Scope11/2
  If/2 -> If Action Subsystem1/Action
  Constant/1 -> Relational Operator/2
  If1/2 -> If Action Subsystem3/Action
  Relational Operator/1 -> Scope4/1, Subsystem2/Trigger, Scope3/1
  Pulse Generator1/1 -> Scope12/1, Discrete-Time Integrator3/2, Subsystem1/Trigger
  Abs/1 -> Scope10/2, Discrete-Time Integrator2/1
  Discrete-Time Integrator3/1 -> Subsystem1/1(In1), Scope13/1
  Merge/1 -> Sin/1, Scope14/1
  If Action Subsystem1/1(Out1) -> Merge/2
  Subsystem1/1(Out1) -> If Action Subsystem3/1(In1), If Action Subsystem2/1(In1), Relational Operator1/1, Scope5/1, Scope16/2, Scope11/1
  If Action Subsystem/1(Out1) -> Merge/1
  If Action Subsystem3/1(Out1) -> Merge1/2
  If/1 -> If Action Subsystem/Action
  Vx/1 -> Abs/1
  Vy/1 -> Abs1/1

== system PMSM_FOC_Tractio/PMSM/SVPWM1 ==
  Tcm1 : Inport
  Tcm2 : Inport  Port=2
  Tcm3 : Inport  Port=3
  carrier : Inport  Port=4
  Add1 : Sum  Inputs=+-
  Add2 : Sum  Inputs=+-
  Add3 : Sum  Inputs=+-
  Bus Creator : BusCreator  Inputs=6
  Data Type Conversion : DataTypeConversion  OutDataTypeStr=double
  Data Type Conversion1 : DataTypeConversion  OutDataTypeStr=double
  Data Type Conversion2 : DataTypeConversion  OutDataTypeStr=double
  Logical Operator : Logic  Operator=NOT  AllPortsSameDT=off  OutDataTypeStr=boolean
  Logical Operator1 : Logic  Operator=NOT  AllPortsSameDT=off  OutDataTypeStr=boolean
  Logical Operator2 : Logic  Operator=NOT  AllPortsSameDT=off  OutDataTypeStr=boolean
  Relay : Relay
  Relay1 : Relay
  Relay2 : Relay
  pulse : Outport
  wires:
  carrier/1 -> Add1/1, Add2/1, Add3/1
  Tcm2/1 -> Add2/2
  Tcm3/1 -> Add3/2
  Add3/1 -> Relay2/1
  Add2/1 -> Relay1/1
  Add1/1 -> Relay/1
  Tcm1/1 -> Add1/2
  Relay2/1 -> Logical Operator2/1, Bus Creator/5
  Relay/1 -> Logical Operator/1, Bus Creator/1
  Relay1/1 -> Logical Operator1/1, Bus Creator/3
  Data Type Conversion2/1 -> Bus Creator/6
  Logical Operator2/1 -> Data Type Conversion2/1
  Data Type Conversion1/1 -> Bus Creator/4
  Logical Operator1/1 -> Data Type Conversion1/1
  Data Type Conversion/1 -> Bus Creator/2
  Logical Operator/1 -> Data Type Conversion/1
  Bus Creator/1 -> pulse/1

== system PMSM_FOC_Tractio/PMSM/W_R ==
  w : Inport
  Angular Velocity Source : fl_lib/Mechanical/Mechanical Sources/Ideal Angular Velocity Source
  Mechanical Rotational Reference2 : fl_lib/Mechanical/Rotational Elements/Mechanical Rotational Reference
  Simulink-PS Converter : nesl_utility/Simulink-PS Converter  PhysicalDomain=network_engine_domain  SubClassName=ps_input  LeftPortType=input  RightPortType=output  PseudoPeriodic=off  Frequencies=[]  NoiseDistribution=none  NoiseParameters=[]  Unit=rad/s  AffineConversion=off  FilteringAndDerivatives=zero  SimscapeFilterOrder=1  InputFilterTimeConstant=0.0001  UdotUserProvided=1
  Torque Sensor : Subsystem
  R : PMIOPort  Side=Right
  C : PMIOPort  Port=2  Side=Right
  tag scope: wref=global
  wires:
  w/1 -> [wref], Simulink-PS Converter/1
  connections:
  Mechanical Rotational Reference2/LConn1 -- C/RConn1 -- Angular Velocity Source/RConn2
  Simulink-PS Converter/RConn1 -- Angular Velocity Source/RConn1
  Torque Sensor/LConn1 -- R/RConn1
  Torque Sensor/RConn1 -- Angular Velocity Source/LConn1
